simulink model "Part_H"  (R2020a)
settings: Solver=FixedStepAuto  StartTime=0.0  StopTime=stop_time  FixedStep=0.1/1000  RelTol=1e-3
values from neighbouring files (symbols this model uses):
  B_x = 0.0094    [Project_3_Prelab.m]
  B_y = 0.0091    [Project_3_Prelab.m]
  Je_x = 4.36E-4    (= 0.000436)    [Project_3_Prelab.m]
  Je_y = 3E-4    (= 0.0003)    [Project_3_Prelab.m]
  Ka = 1    [Project_3_Prelab.m]
  Ke = 1.59    [Project_3_Prelab.m]
  Kt = 0.49    [Project_3_Prelab.m]
  R_x_Z = 1+r1*z^-1    [Project_3_Prelab.m]
  R_y_Z = R_y_Z_mytraj    [Project_3_Lab.m]    (also in Project_3_Prelab.m = 1+r1*z^-1)
libraries: cstblocks x6, simulink x1
settings Model: Creator=jchia  LastModifiedBy=jchia

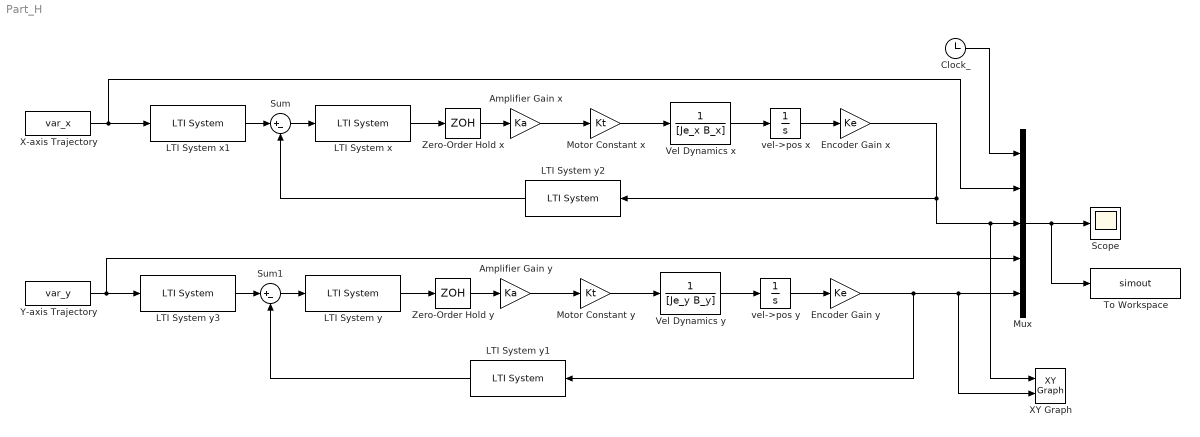
== system Part_H ==
  Amplifier Gain x : Gain  Gain=Ka
  Amplifier Gain y : Gain  Gain=Ka
  Clock_ : Clock
  Encoder Gain x : Gain  Gain=Ke
  Encoder Gain y : Gain  Gain=Ke
  LTI System x : cstblocks/LTI System  sys=1/R_x_Z  IC=[]
  LTI System x1 : cstblocks/LTI System  sys=t0_x_Z  IC=[]
  LTI System y : cstblocks/LTI System  sys=1/R_y_Z  IC=[]
  LTI System y1 : cstblocks/LTI System  sys=s_y_Z  IC=[]
  LTI System y2 : cstblocks/LTI System  sys=s_x_Z  IC=[]
  LTI System y3 : cstblocks/LTI System  sys=t0_y_Z  IC=[]
  Motor Constant x : Gain  Gain=Kt
  Motor Constant y : Gain  Gain=Kt
  Mux : Mux  Inputs=5
  Scope : Scope
  Sum : Sum  Inputs=|+-
  Sum1 : Sum  Inputs=|+-
  To Workspace : ToWorkspace  VariableName=simout  SaveFormat=Structure With Time  SampleTime=-1
  Vel Dynamics x : TransferFcn  Denominator=[Je_x B_x]
  Vel Dynamics y : TransferFcn  Denominator=[Je_y B_y]
  X-axis Trajectory : FromWorkspace  VariableName=var_x
  "XY Graph " : simulink/Sinks/XY Graph  xmin=0  xmax=125  ymin=-5  ymax=85  st=-1
  Y-axis Trajectory : FromWorkspace  VariableName=var_y
  Zero-Order Hold x : ZeroOrderHold  SampleTime=-1
  Zero-Order Hold y : ZeroOrderHold  SampleTime=-1
  vel->pos x : Integrator
  vel->pos y : Integrator
  wires:
  Vel Dynamics y/1 -> vel->pos y/1
  Mux/1 -> To Workspace/1, Scope/1
  Zero-Order Hold y/1 -> Amplifier Gain y/1
  Y-axis Trajectory/1 -> LTI System y3/1, Mux/4
  vel->pos y/1 -> Encoder Gain y/1
  Amplifier Gain y/1 -> Motor Constant y/1
  Encoder Gain x/1 -> LTI System y2/1, "XY Graph "/1, Mux/3
  Motor Constant y/1 -> Vel Dynamics y/1
  Zero-Order Hold x/1 -> Amplifier Gain x/1
  vel->pos x/1 -> Encoder Gain x/1
  Sum/1 -> LTI System x/1
  LTI System y/1 -> Zero-Order Hold y/1
  Amplifier Gain x/1 -> Motor Constant x/1
  Encoder Gain y/1 -> LTI System y1/1, "XY Graph "/2, Mux/5
  Clock_/1 -> Mux/1
  Vel Dynamics x/1 -> vel->pos x/1
  Motor Constant x/1 -> Vel Dynamics x/1
  X-axis Trajectory/1 -> LTI System x1/1, Mux/2
  LTI System x/1 -> Zero-Order Hold x/1
  Sum1/1 -> LTI System y/1
  LTI System y1/1 -> Sum1/2
  LTI System y2/1 -> Sum/2
  LTI System x1/1 -> Sum/1
  LTI System y3/1 -> Sum1/1
